simulink model "bh_motor_just_dc_motor_EXPLORE"  (R2017b)
settings: Solver=ode15s  StartTime=0.0  StopTime=30  RelTol=1e-3  EnableMultiTasking=on
undefined symbols (not defined in the file): sigbuilder_block
libraries: fl_lib x30, nesl_utility x20, elec_lib x3
settings Model: Creator=bhorton  LastModifiedBy=bhorton
settings DataIOCC: LimitDataPoints=on
settings OptimizationCC: LifeSpan=inf
settings DebuggingCC: AllowSymbolicDim=off  SFUnexpectedBacktrackingDiag=warning  SFNoUnconditionalDefaultTransitionDiag=warning  SFExecutionAtInitializationDiag=none
settings ModelReferenceCC: PropagateSignalLabelsOutOfModel=off
settings CodeAppCC: StateflowObjectComments=on
settings GRTTargetCC: TargetLangStandard=C89/C90 (ANSI)
settings ConfigComp: CovMetricSettings=dw  CovHtmlReporting=on  CovSaveCumulativeToWorkspaceVar=on  CovSaveSingleToWorkspaceVar=on  CovExternalEMLEnable=off
settings SimscapeCC: SimscapeNormalizeSystem=off  SimscapeLogType=all  SimscapeLogDataHistory=10000  SelectedTab=SimMechanics

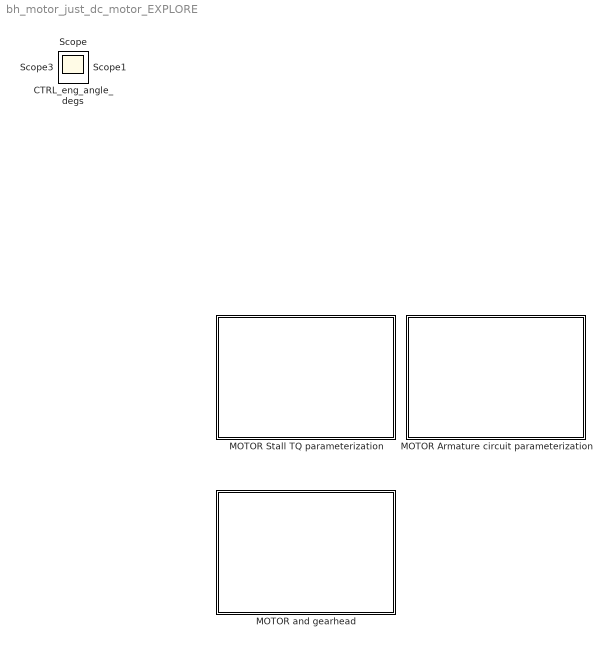
== system bh_motor_just_dc_motor_EXPLORE ==
  MOTOR Armature circuit parameterization : Subsystem
  MOTOR Stall TQ parameterization : Subsystem
  MOTOR and gearhead : Subsystem
  CTRL_eng_angle_degs : Scope
  Scope : Scope
  Scope1 : Scope
  Scope3 : Scope

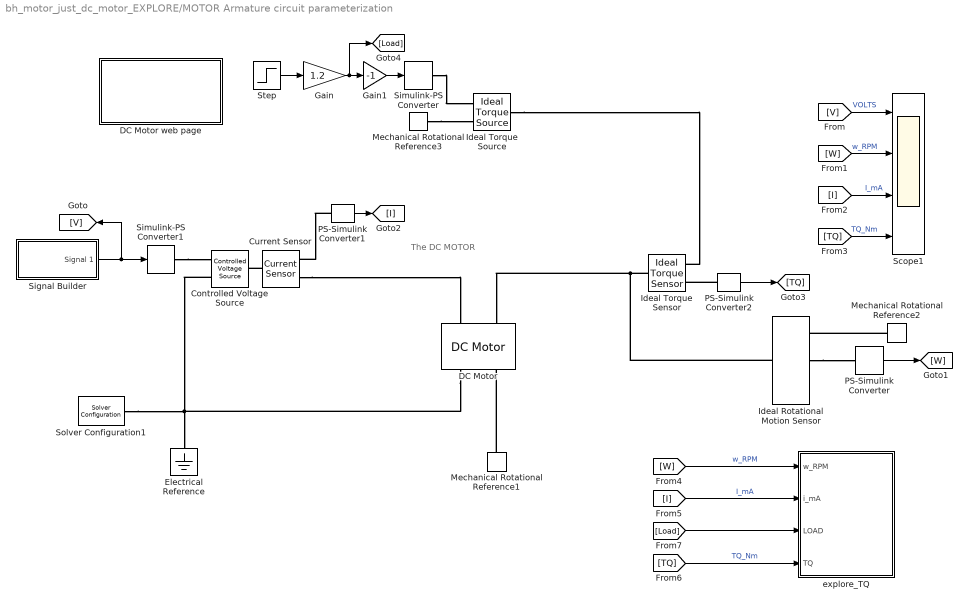
== system bh_motor_just_dc_motor_EXPLORE/MOTOR Armature circuit parameterization ==
  note: The DC MOTOR
  Controlled Voltage Source : fl_lib/Electrical/Electrical Sources/Controlled Voltage Source
  Current Sensor : fl_lib/Electrical/Electrical Sensors/Current Sensor
  DC Motor : elec_lib/Actuators & Drivers/Rotational Actuators/DC Motor  parameterization=1  Ra=5.0117 Ohm  La=1e-4 H  emf_or_torque=2  Kv=7.2e-5 V/rpm  Ki=0.57296 *0.875 N*m/A  T_stall=1.2 N*m  w_max=200 rpm  w_rated=1.5e+4 rpm  P_rated=0.08 W  V_rated=12 V  J=4.5e-5 kg*m^2  lam_param=1  lam=8.20705e-3 N*m/(rad/s)  i_noload=300 mA  V_i_noload=12 V  speed0=0 rpm  alpha=0.00393 1/K  Tmeas=25 C  thermal_mass=100 J/K  initial_temperature=25 C
  DC Motor web page : Subsystem
  Electrical Reference : fl_lib/Electrical/Electrical Elements/Electrical Reference
  Gain : Gain  Gain=1.2
  Gain1 : Gain  Gain=-1
  Ideal Rotational Motion Sensor : fl_lib/Mechanical/Mechanical Sensors/Ideal Rotational Motion Sensor  offset=0 rad
  Ideal Torque Sensor : fl_lib/Mechanical/Mechanical Sensors/Ideal Torque Sensor
  Ideal Torque Source : fl_lib/Mechanical/Mechanical Sources/Ideal Torque Source
  Mechanical Rotational Reference1 : fl_lib/Mechanical/Rotational Elements/Mechanical Rotational Reference
  Mechanical Rotational Reference2 : fl_lib/Mechanical/Rotational Elements/Mechanical Rotational Reference
  Mechanical Rotational Reference3 : fl_lib/Mechanical/Rotational Elements/Mechanical Rotational Reference
  PS-Simulink Converter : nesl_utility/PS-Simulink Converter  PhysicalDomain=network_engine_domain  SubClassName=ps_output  LeftPortType=input  RightPortType=output  PseudoPeriodic=off  Frequencies=[]  Unit=rpm  AffineConversion=off
  PS-Simulink Converter1 : nesl_utility/PS-Simulink Converter  PhysicalDomain=network_engine_domain  SubClassName=ps_output  LeftPortType=input  RightPortType=output  PseudoPeriodic=off  Frequencies=[]  Unit=mA  AffineConversion=off
  PS-Simulink Converter2 : nesl_utility/PS-Simulink Converter  PhysicalDomain=network_engine_domain  SubClassName=ps_output  LeftPortType=input  RightPortType=output  PseudoPeriodic=off  Frequencies=[]  Unit=N*m  AffineConversion=off
  Scope1 : Scope  NumInputPorts=4
  Signal Builder : Subsystem  Tag=STV Subsys  LoadFcn=sigbuilder_block('load');  StartFcn=sigbuilder_block('start');  StopFcn=sigbuilder_block('stop');  ClipboardFcn=sigbuilder_block('clipboard');  mask(Sigbuilder block){tuvar=[0:10]}
      mask help: Simulink:masks:SigbuilderBlock_MD
      mask init:
      | if ~strcmp(get_param(bdroot(gcbh),'SimulationStatus'),'stopped') tuvar = sigbuilder_block('maskInit'); end
      settings: CopyFcn=sigbuilder_block('copy');  DeleteFcn=sigbuilder_block('delete');  ModelCloseFcn=sigbuilder_block('modelClose');  PreSaveFcn=sigbuilder_block('preSave');  PauseFcn=sigbuilder_block('pause');  ContinueFcn=sigbuilder_block('continue');  NameChangeFcn=sigbuilder_block('namechange');  OpenFcn=sigbuilder_block('open',[437.6 199.2 550.4 400 ]);  CloseFcn=sigbuilder_block('close');
      mask Display: plot(0, 0, 100, 100,[2, 2, 32, 32, 2], [68, 8, 8, 68, 68],[32, 2], [38, 38], [32, 19, 2],[53, 60, 44], [32, 17, 17, 2],[16, 16, 31, 31]);txt = getActiveGroup(gcbh);text(2, 100, txt,'verticalAlignment', 'top');
  Simulink-PS Converter : nesl_utility/Simulink-PS Converter  PhysicalDomain=network_engine_domain  SubClassName=ps_input  LeftPortType=input  RightPortType=output  PseudoPeriodic=off  Frequencies=[]  NoiseDistribution=none  NoiseParameters=[]  Unit=N*m  AffineConversion=off  FilteringAndDerivatives=provide  SimscapeFilterOrder=1  InputFilterTimeConstant=0.001  UdotUserProvided=0
  Simulink-PS Converter1 : nesl_utility/Simulink-PS Converter  PhysicalDomain=network_engine_domain  SubClassName=ps_input  LeftPortType=input  RightPortType=output  PseudoPeriodic=off  Frequencies=[]  NoiseDistribution=none  NoiseParameters=[]  Unit=V  AffineConversion=off  FilteringAndDerivatives=zero  SimscapeFilterOrder=1  InputFilterTimeConstant=0.001  UdotUserProvided=1
  Solver Configuration1 : nesl_utility/Solver Configuration  PhysicalDomain=network_engine_domain  SubClassName=solver  LeftPortType=input  RightPortType=generic  Accelerate=off  Tones=[]  Harmonics=[]  SimulateNoise=off  Profile=off  UseLocalSampling=off  EnableSwitchedLinearOptims=on  FrequencyDomain=off  UseCCode=off  RelTol=0.001  AbsTol=1e-06  MinStep=1e-09  ToWorkspace=off  RevertToSquareIcSolve=off  NumHomotopyIterations=100  PhasorMode=off  PhasorModeNumHarmonics=1  DoDC=off  ResidualTolerance=1e-09  UseLocalSolver=off  LocalSolverChoice=NE_BACKWARD_EULER_ADVANCER  LocalSolverSampleTime=0.001  DoFixedCost=off  MaxNonlinIter=3  MaxModeIter=2  LinearAlgebra=Sparse  DelaysMemoryBudget=1024  AutomaticFiltering=on  FilteringTimeConstant=0.001
  Step : Step  Time=25  SampleTime=0
      settings: AttributesFormatString=Step @ t= %<Time>
  explore_TQ : Subsystem
  wires:
  PS-Simulink Converter1/1 -> [I]
  Signal Builder/1(Signal 1) -> [V], Simulink-PS Converter1/1
  [V] -> Scope1/1  "VOLTS"
  [W] -> Scope1/2  "w_RPM"
  [I] -> Scope1/3  "I_mA"
  Step/1 -> Gain/1
  Gain/1 -> [Load], Gain1/1
  PS-Simulink Converter/1 -> [W]
  PS-Simulink Converter2/1 -> [TQ]
  [TQ] -> Scope1/4  "TQ_Nm"
  [TQ] -> explore_TQ/4(TQ)  "TQ_Nm"
  [W] -> explore_TQ/1(w_RPM)  "w_RPM"
  [I] -> explore_TQ/2(i_mA)  "I_mA"
  [Load] -> explore_TQ/3(LOAD)
  Gain1/1 -> Simulink-PS Converter/1
  connections:
  Mechanical Rotational Reference1/LConn1 -- DC Motor/RConn2
  Ideal Rotational Motion Sensor/RConn2 -- PS-Simulink Converter/LConn1
  Mechanical Rotational Reference3/LConn1 -- Ideal Torque Source/RConn2
  Simulink-PS Converter/RConn1 -- Ideal Torque Source/RConn1
  Ideal Torque Source/LConn1 -- Ideal Torque Sensor/RConn1
  Simulink-PS Converter1/RConn1 -- Controlled Voltage Source/RConn1
  Ideal Torque Sensor/LConn1 -- Ideal Rotational Motion Sensor/LConn1 -- DC Motor/LConn2
  Mechanical Rotational Reference2/LConn1 -- Ideal Rotational Motion Sensor/RConn1
  PS-Simulink Converter2/LConn1 -- Ideal Torque Sensor/RConn2
  Controlled Voltage Source/RConn2 -- DC Motor/RConn1 -- Electrical Reference/LConn1 -- Solver Configuration1/RConn1
  PS-Simulink Converter1/LConn1 -- Current Sensor/RConn1
  Current Sensor/RConn2 -- DC Motor/LConn1
  Current Sensor/LConn1 -- Controlled Voltage Source/LConn1

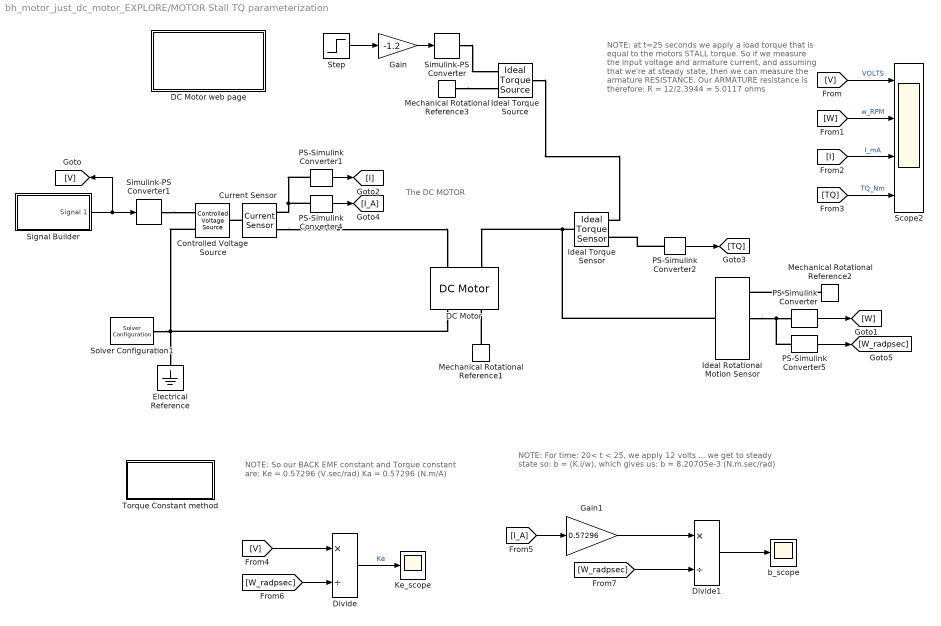
== system bh_motor_just_dc_motor_EXPLORE/MOTOR Stall TQ parameterization ==
  note: The DC MOTOR
  note: NOTE:
      | at t=25 seconds we apply a load torque
      | that is equal to the motors STALL torque.
      |
      | So if we measure the input voltage and armature
      | current, and assuming that we're at steady state,
      | then we can measure the armature RESISTANCE.
      |
      | Our ARMATURE resistance is therefore:
      | R = 12/2.3944 = 5.0117 ohms
  note: NOTE:
      | So our BACK EMF constant and Torque constant are:
      | Ke =  0.57296  (V.sec/rad)
      | Ka =  0.57296  (N.m/A)
  note: NOTE:
      | For time:  20< t < 25, we apply 12 volts ... we get to steady state
      | so:   b = (K.i/w), which gives us:
      | b = 8.20705e-3 (N.m.sec/rad)
  Controlled Voltage Source : fl_lib/Electrical/Electrical Sources/Controlled Voltage Source
  Current Sensor : fl_lib/Electrical/Electrical Sensors/Current Sensor
  DC Motor : elec_lib/Actuators & Drivers/Rotational Actuators/DC Motor  parameterization=2  Ra=2 Ohm  La=1e-4 H  emf_or_torque=2  Kv=7.2e-5 V/rpm  Ki=0.0083 N*m/A  T_stall=1.2 N*m  w_max=200 rpm  w_rated=1.5e+4 rpm  P_rated=0.08 W  V_rated=12 V  J=4.5e-5 kg*m^2  lam_param=2  lam=0.7e-5 N*m/(rad/s)  i_noload=300 mA  V_i_noload=12 V  speed0=0 rpm  alpha=0.00393 1/K  Tmeas=25 C  thermal_mass=100 J/K  initial_temperature=25 C
  DC Motor web page : Subsystem
  Divide : Product  Inputs=*/
  Divide1 : Product  Inputs=*/
  Electrical Reference : fl_lib/Electrical/Electrical Elements/Electrical Reference
  Gain : Gain  Gain=-1.2
  Gain1 : Gain  Gain=0.57296
  Ideal Rotational Motion Sensor : fl_lib/Mechanical/Mechanical Sensors/Ideal Rotational Motion Sensor  offset=0 rad
  Ideal Torque Sensor : fl_lib/Mechanical/Mechanical Sensors/Ideal Torque Sensor
  Ideal Torque Source : fl_lib/Mechanical/Mechanical Sources/Ideal Torque Source
  Ke_scope : Scope
  Mechanical Rotational Reference1 : fl_lib/Mechanical/Rotational Elements/Mechanical Rotational Reference
  Mechanical Rotational Reference2 : fl_lib/Mechanical/Rotational Elements/Mechanical Rotational Reference
  Mechanical Rotational Reference3 : fl_lib/Mechanical/Rotational Elements/Mechanical Rotational Reference
  PS-Simulink Converter : nesl_utility/PS-Simulink Converter  PhysicalDomain=network_engine_domain  SubClassName=ps_output  LeftPortType=input  RightPortType=output  PseudoPeriodic=off  Frequencies=[]  Unit=rpm  AffineConversion=off
  PS-Simulink Converter1 : nesl_utility/PS-Simulink Converter  PhysicalDomain=network_engine_domain  SubClassName=ps_output  LeftPortType=input  RightPortType=output  PseudoPeriodic=off  Frequencies=[]  Unit=mA  AffineConversion=off
  PS-Simulink Converter2 : nesl_utility/PS-Simulink Converter  PhysicalDomain=network_engine_domain  SubClassName=ps_output  LeftPortType=input  RightPortType=output  PseudoPeriodic=off  Frequencies=[]  Unit=N*m  AffineConversion=off
  PS-Simulink Converter4 : nesl_utility/PS-Simulink Converter  PhysicalDomain=network_engine_domain  SubClassName=ps_output  LeftPortType=input  RightPortType=output  PseudoPeriodic=off  Frequencies=[]  Unit=A  AffineConversion=off
  PS-Simulink Converter5 : nesl_utility/PS-Simulink Converter  PhysicalDomain=network_engine_domain  SubClassName=ps_output  LeftPortType=input  RightPortType=output  PseudoPeriodic=off  Frequencies=[]  Unit=rad/s  AffineConversion=off
  Scope2 : Scope  NumInputPorts=4
  Signal Builder : Subsystem  Tag=STV Subsys  LoadFcn=sigbuilder_block('load');  StartFcn=sigbuilder_block('start');  StopFcn=sigbuilder_block('stop');  ClipboardFcn=sigbuilder_block('clipboard');  mask(Sigbuilder block){tuvar=[0:10]}
      mask help: Simulink:masks:SigbuilderBlock_MD
      mask init:
      | if ~strcmp(get_param(bdroot(gcbh),'SimulationStatus'),'stopped') tuvar = sigbuilder_block('maskInit'); end
      settings: CopyFcn=sigbuilder_block('copy');  DeleteFcn=sigbuilder_block('delete');  ModelCloseFcn=sigbuilder_block('modelClose');  PreSaveFcn=sigbuilder_block('preSave');  PauseFcn=sigbuilder_block('pause');  ContinueFcn=sigbuilder_block('continue');  NameChangeFcn=sigbuilder_block('namechange');  OpenFcn=sigbuilder_block('open',[437.6 199.2 550.4 400 ]);  CloseFcn=sigbuilder_block('close');
      mask Display: plot(0, 0, 100, 100,[2, 2, 32, 32, 2], [68, 8, 8, 68, 68],[32, 2], [38, 38], [32, 19, 2],[53, 60, 44], [32, 17, 17, 2],[16, 16, 31, 31]);txt = getActiveGroup(gcbh);text(2, 100, txt,'verticalAlignment', 'top');
  Simulink-PS Converter : nesl_utility/Simulink-PS Converter  PhysicalDomain=network_engine_domain  SubClassName=ps_input  LeftPortType=input  RightPortType=output  PseudoPeriodic=off  Frequencies=[]  NoiseDistribution=none  NoiseParameters=[]  Unit=N*m  AffineConversion=off  FilteringAndDerivatives=provide  SimscapeFilterOrder=1  InputFilterTimeConstant=0.001  UdotUserProvided=0
  Simulink-PS Converter1 : nesl_utility/Simulink-PS Converter  PhysicalDomain=network_engine_domain  SubClassName=ps_input  LeftPortType=input  RightPortType=output  PseudoPeriodic=off  Frequencies=[]  NoiseDistribution=none  NoiseParameters=[]  Unit=V  AffineConversion=off  FilteringAndDerivatives=zero  SimscapeFilterOrder=1  InputFilterTimeConstant=0.001  UdotUserProvided=1
  Solver Configuration1 : nesl_utility/Solver Configuration  PhysicalDomain=network_engine_domain  SubClassName=solver  LeftPortType=input  RightPortType=generic  Accelerate=off  Tones=[]  Harmonics=[]  SimulateNoise=off  Profile=off  UseLocalSampling=off  EnableSwitchedLinearOptims=on  FrequencyDomain=off  UseCCode=off  RelTol=0.001  AbsTol=1e-06  MinStep=1e-09  ToWorkspace=off  RevertToSquareIcSolve=off  NumHomotopyIterations=100  PhasorMode=off  PhasorModeNumHarmonics=1  DoDC=off  ResidualTolerance=1e-09  UseLocalSolver=off  LocalSolverChoice=NE_BACKWARD_EULER_ADVANCER  LocalSolverSampleTime=0.001  DoFixedCost=off  MaxNonlinIter=3  MaxModeIter=2  LinearAlgebra=Sparse  DelaysMemoryBudget=1024  AutomaticFiltering=on  FilteringTimeConstant=0.001
  Step : Step  Time=25  SampleTime=0
      settings: AttributesFormatString=Step @ t= %<Time>
  Torque Constant method : Subsystem
  b_scope : Scope
  wires:
  PS-Simulink Converter1/1 -> [I]
  Signal Builder/1(Signal 1) -> [V], Simulink-PS Converter1/1
  [V] -> Scope2/1  "VOLTS"
  [W] -> Scope2/2  "w_RPM"
  [I] -> Scope2/3  "I_mA"
  Step/1 -> Gain/1
  Gain/1 -> Simulink-PS Converter/1
  PS-Simulink Converter/1 -> [W]
  PS-Simulink Converter2/1 -> [TQ]
  [TQ] -> Scope2/4  "TQ_Nm"
  [V] -> Divide/1
  Divide/1 -> Ke_scope/1  "Ke"
  PS-Simulink Converter4/1 -> [I_A]
  [I_A] -> Gain1/1
  Gain1/1 -> Divide1/1
  PS-Simulink Converter5/1 -> [W_radpsec]
  [W_radpsec] -> Divide/2
  [W_radpsec] -> Divide1/2
  Divide1/1 -> b_scope/1
  connections:
  Mechanical Rotational Reference1/LConn1 -- DC Motor/RConn2
  Ideal Rotational Motion Sensor/RConn2 -- PS-Simulink Converter5/LConn1 -- PS-Simulink Converter/LConn1
  Mechanical Rotational Reference3/LConn1 -- Ideal Torque Source/RConn2
  Simulink-PS Converter/RConn1 -- Ideal Torque Source/RConn1
  Ideal Torque Source/LConn1 -- Ideal Torque Sensor/RConn1
  Simulink-PS Converter1/RConn1 -- Controlled Voltage Source/RConn1
  Ideal Torque Sensor/LConn1 -- Ideal Rotational Motion Sensor/LConn1 -- DC Motor/LConn2
  Mechanical Rotational Reference2/LConn1 -- Ideal Rotational Motion Sensor/RConn1
  PS-Simulink Converter2/LConn1 -- Ideal Torque Sensor/RConn2
  Controlled Voltage Source/RConn2 -- DC Motor/RConn1 -- Electrical Reference/LConn1 -- Solver Configuration1/RConn1
  PS-Simulink Converter1/LConn1 -- PS-Simulink Converter4/LConn1 -- Current Sensor/RConn1
  Current Sensor/RConn2 -- DC Motor/LConn1
  Current Sensor/LConn1 -- Controlled Voltage Source/LConn1

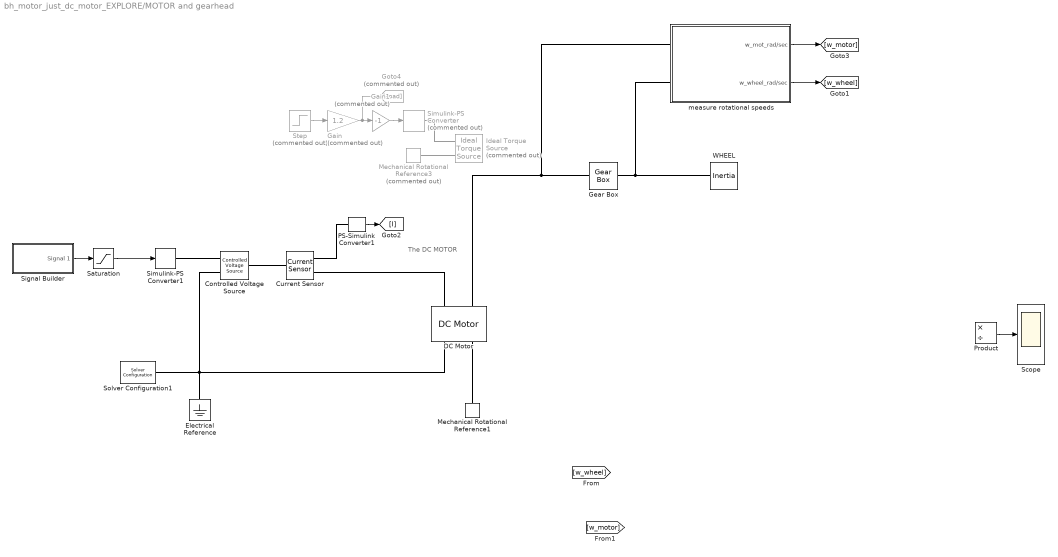
== system bh_motor_just_dc_motor_EXPLORE/MOTOR and gearhead ==
  note: The DC MOTOR
  Controlled Voltage Source : fl_lib/Electrical/Electrical Sources/Controlled Voltage Source
  Current Sensor : fl_lib/Electrical/Electrical Sensors/Current Sensor
  DC Motor : elec_lib/Actuators & Drivers/Rotational Actuators/DC Motor  parameterization=1  Ra=5.0117 Ohm  La=1e-4 H  emf_or_torque=2  Kv=7.2e-5 V/rpm  Ki=0.57296 *0.875 N*m/A  T_stall=1.2 N*m  w_max=200 rpm  w_rated=1.5e+4 rpm  P_rated=0.08 W  V_rated=12 V  J=4.5e-5 kg*m^2  lam_param=1  lam=8.20705e-3 N*m/(rad/s)  i_noload=300 mA  V_i_noload=12 V  speed0=0 rpm  alpha=0.00393 1/K  Tmeas=25 C  thermal_mass=100 J/K  initial_temperature=25 C
  Electrical Reference : fl_lib/Electrical/Electrical Elements/Electrical Reference
  Gain : Gain  Commented=on  Gain=1.2
  Gain1 : Gain  Commented=on  Gain=-1
  Gear Box : fl_lib/Mechanical/Mechanisms/Gear Box  ratio=1  t_in_specify=off  t_in_priority=None  t_in=0 N*m  t_in_nominal_specify=off  t_in_nominal_unit=N*m  t_in_nominal_value=1  t_out_specify=off  t_out_priority=None  t_out=0 N*m  t_out_nominal_specify=off  t_out_nominal_unit=N*m  t_out_nominal_value=1
      settings: AttributesFormatString=|
      | G = (w_in     / w_out)
      | G = (T_out /  T_in)
      | G = %<ratio>
  Goto4 : Goto  Commented=on  GotoTag=Load
  Ideal Torque Source : fl_lib/Mechanical/Mechanical Sources/Ideal Torque Source  Commented=on
  Mechanical Rotational Reference1 : fl_lib/Mechanical/Rotational Elements/Mechanical Rotational Reference
  Mechanical Rotational Reference3 : fl_lib/Mechanical/Rotational Elements/Mechanical Rotational Reference  Commented=on
  PS-Simulink Converter1 : nesl_utility/PS-Simulink Converter  PhysicalDomain=network_engine_domain  SubClassName=ps_output  LeftPortType=input  RightPortType=output  PseudoPeriodic=off  Frequencies=[]  Unit=mA  AffineConversion=off
  Product : Product  Inputs=*/
  Saturation : Saturate
  Scope : Scope  NumInputPorts=3
  Signal Builder : Subsystem  Tag=STV Subsys  LoadFcn=sigbuilder_block('load');  StartFcn=sigbuilder_block('start');  StopFcn=sigbuilder_block('stop');  ClipboardFcn=sigbuilder_block('clipboard');  mask(Sigbuilder block){tuvar=[0:10]}
      mask help: Simulink:masks:SigbuilderBlock_MD
      mask init:
      | if ~strcmp(get_param(bdroot(gcbh),'SimulationStatus'),'stopped') tuvar = sigbuilder_block('maskInit'); end
      settings: CopyFcn=sigbuilder_block('copy');  DeleteFcn=sigbuilder_block('delete');  ModelCloseFcn=sigbuilder_block('modelClose');  PreSaveFcn=sigbuilder_block('preSave');  PauseFcn=sigbuilder_block('pause');  ContinueFcn=sigbuilder_block('continue');  NameChangeFcn=sigbuilder_block('namechange');  OpenFcn=sigbuilder_block('open',[437.6 199.2 550.4 400 ]);  CloseFcn=sigbuilder_block('close');
      mask Display: plot(0, 0, 100, 100,[2, 2, 32, 32, 2], [68, 8, 8, 68, 68],[32, 2], [38, 38], [32, 19, 2],[53, 60, 44], [32, 17, 17, 2],[16, 16, 31, 31]);txt = getActiveGroup(gcbh);text(2, 100, txt,'verticalAlignment', 'top');
  Simulink-PS Converter : nesl_utility/Simulink-PS Converter  Commented=on  PhysicalDomain=network_engine_domain  SubClassName=ps_input  LeftPortType=input  RightPortType=output  PseudoPeriodic=off  Frequencies=[]  NoiseDistribution=none  NoiseParameters=[]  Unit=N*m  AffineConversion=off  FilteringAndDerivatives=provide  SimscapeFilterOrder=1  InputFilterTimeConstant=0.001  UdotUserProvided=0
  Simulink-PS Converter1 : nesl_utility/Simulink-PS Converter  PhysicalDomain=network_engine_domain  SubClassName=ps_input  LeftPortType=input  RightPortType=output  PseudoPeriodic=off  Frequencies=[]  NoiseDistribution=none  NoiseParameters=[]  Unit=V  AffineConversion=off  FilteringAndDerivatives=zero  SimscapeFilterOrder=1  InputFilterTimeConstant=0.001  UdotUserProvided=1
  Solver Configuration1 : nesl_utility/Solver Configuration  PhysicalDomain=network_engine_domain  SubClassName=solver  LeftPortType=input  RightPortType=generic  Accelerate=off  Tones=[]  Harmonics=[]  SimulateNoise=off  Profile=off  UseLocalSampling=off  EnableSwitchedLinearOptims=on  FrequencyDomain=off  UseCCode=off  RelTol=0.001  AbsTol=1e-06  MinStep=1e-09  ToWorkspace=off  RevertToSquareIcSolve=off  NumHomotopyIterations=100  PhasorMode=off  PhasorModeNumHarmonics=1  DoDC=off  ResidualTolerance=1e-09  UseLocalSolver=off  LocalSolverChoice=NE_BACKWARD_EULER_ADVANCER  LocalSolverSampleTime=0.001  DoFixedCost=off  MaxNonlinIter=3  MaxModeIter=2  LinearAlgebra=Sparse  DelaysMemoryBudget=1024  AutomaticFiltering=on  FilteringTimeConstant=0.001
  Step : Step  Commented=on  Time=25  SampleTime=0
      settings: AttributesFormatString=Step @ t= %<Time>
  WHEEL : fl_lib/Mechanical/Rotational Elements/Inertia  inertia=0.01 kg*m^2  w_specify=off  w_priority=High  w=0 rad/s  w_nominal_specify=off  w_nominal_unit=rad/s  w_nominal_value=1  t_specify=off  t_priority=None  t=0 N*m  t_nominal_specify=off  t_nominal_unit=N*m  t_nominal_value=1
  measure rotational speeds : Subsystem
  wires:
  PS-Simulink Converter1/1 -> [I]
  Signal Builder/1(Signal 1) -> Saturation/1
  Step/1 -> Gain/1
  Gain/1 -> Goto4/1, Gain1/1
  Gain1/1 -> Simulink-PS Converter/1
  Product/1 -> Scope/2
  Saturation/1 -> Simulink-PS Converter1/1
  measure rotational speeds/2(w_wheel_rad/sec) -> [w_wheel]
  measure rotational speeds/1(w_mot_rad/sec) -> [w_motor]
  connections:
  Mechanical Rotational Reference1/LConn1 -- DC Motor/RConn2
  Mechanical Rotational Reference3/LConn1 -- Ideal Torque Source/RConn2
  Simulink-PS Converter/RConn1 -- Ideal Torque Source/RConn1
  Simulink-PS Converter1/RConn1 -- Controlled Voltage Source/RConn1
  Controlled Voltage Source/RConn2 -- DC Motor/RConn1 -- Solver Configuration1/RConn1 -- Electrical Reference/LConn1
  PS-Simulink Converter1/LConn1 -- Current Sensor/RConn1
  Current Sensor/RConn2 -- DC Motor/LConn1
  Current Sensor/LConn1 -- Controlled Voltage Source/LConn1
  Gear Box/LConn1 -- measure rotational speeds/LConn1 -- DC Motor/LConn2
  WHEEL/LConn1 -- measure rotational speeds/LConn2 -- Gear Box/RConn1

== system bh_motor_just_dc_motor_EXPLORE/MOTOR Armature circuit parameterization/DC Motor web page ==
  note: http://www.onlineconversion.com/torque.htm
  note: 170 ounce inch = 1.2004638117 newton meter
  note: 50:1 powerful brushed DC motor
      | Speed (no load): 200RPM (12V)
      | Stall torque: 170 oz·in (12V)
      | Free-run current (no load): 300 mA (12V)
  note: http://www.robotshop.com/en/12v-501-170oz-inc-metal-gearmotor.html

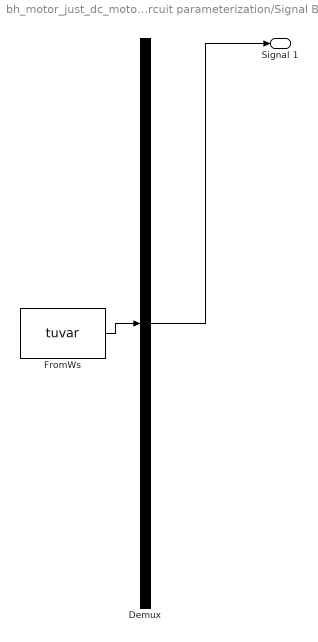
== system bh_motor_just_dc_motor_EXPLORE/MOTOR Armature circuit parameterization/Signal Builder ==
  Demux : Demux  Tag=STV Demux  Outputs=1
  FromWs : FromWorkspace  Tag=STV FromWs  VariableName=tuvar  SampleTime=0
      SigBuilderData=|
      | common.afterFinalStr = 'Extrapolate'
      | common.sampleTime = 0
      | dataSet.timeRange = [0 30]
      | dataSet.name = 'Group 1'
      | sbobj.Groups.Name = 'Group 1'
      | sbobj.Groups.Signals.Name = 'Signal 1'
      | sbobj.Groups.Signals.XData = [0 5.05 5.05 10 10 15.05 15.05 20 20 24.95 30]
      | sbobj.Groups.Signals.YData = [1 1 3 3 6 6 9 9 12 12 12]
      | sbobj.Groups.TimeRange = [0 30]
  Signal 1 : Outport  Tag=STV Outport
  wires:
  Demux/1 -> Signal 1/1
  FromWs/1 -> Demux/1

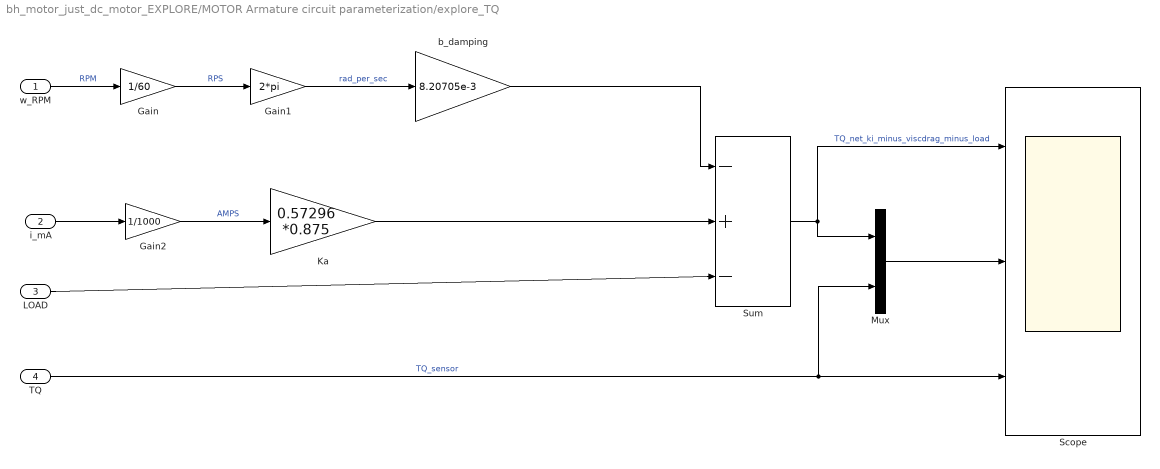
== system bh_motor_just_dc_motor_EXPLORE/MOTOR Armature circuit parameterization/explore_TQ ==
  w_RPM : Inport
  i_mA : Inport  Port=2
  LOAD : Inport  Port=3
  TQ : Inport  Port=4
  Gain : Gain  Gain=1/60
  Gain1 : Gain  Gain=2*pi
  Gain2 : Gain  Gain=1/1000
  Ka : Gain  Gain=0.57296 *0.875
  Mux : Mux  Inputs=2
  Scope : Scope  NumInputPorts=3
  Sum : Sum  Inputs=-|+|-
  b_damping : Gain  Gain=8.20705e-3
  wires:
  w_RPM/1 -> Gain/1  "RPM"
  Gain/1 -> Gain1/1  "RPS"
  Gain1/1 -> b_damping/1  "rad_per_sec"
  i_mA/1 -> Gain2/1
  b_damping/1 -> Sum/1
  Ka/1 -> Sum/2
  Sum/1 -> Scope/1, Mux/1  "TQ_net_ki_minus_viscdrag_minus_load"
  TQ/1 -> Scope/3, Mux/2  "TQ_sensor"
  Gain2/1 -> Ka/1  "AMPS"
  Mux/1 -> Scope/2
  LOAD/1 -> Sum/3

== system bh_motor_just_dc_motor_EXPLORE/MOTOR Stall TQ parameterization/DC Motor web page ==
  note: http://www.onlineconversion.com/torque.htm
  note: 170 ounce inch = 1.2004638117 newton meter
  note: 50:1 powerful brushed DC motor
      | Speed (no load): 200RPM (12V)
      | Stall torque: 170 oz·in (12V)
      | Free-run current (no load): 300 mA (12V)
  note: http://www.robotshop.com/en/12v-501-170oz-inc-metal-gearmotor.html

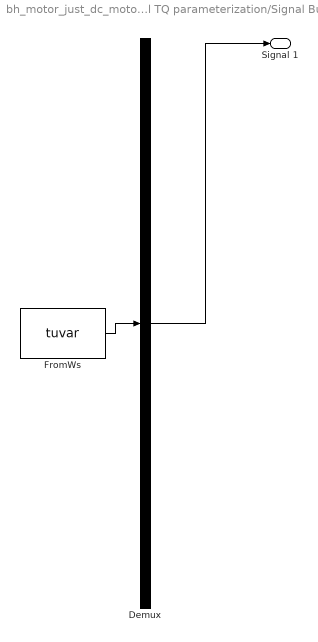
== system bh_motor_just_dc_motor_EXPLORE/MOTOR Stall TQ parameterization/Signal Builder ==
  Demux : Demux  Tag=STV Demux  Outputs=1
  FromWs : FromWorkspace  Tag=STV FromWs  VariableName=tuvar  SampleTime=0
      SigBuilderData=|
      | common.afterFinalStr = 'Extrapolate'
      | common.sampleTime = 0
      | dataSet.timeRange = [0 30]
      | dataSet.name = 'Group 1'
      | sbobj.Groups.Name = 'Group 1'
      | sbobj.Groups.Signals.Name = 'Signal 1'
      | sbobj.Groups.Signals.XData = [0 5.05 5.05 10 10 15.05 15.05 20 20 24.95 30]
      | sbobj.Groups.Signals.YData = [1 1 3 3 6 6 9 9 12 12 12]
      | sbobj.Groups.TimeRange = [0 30]
  Signal 1 : Outport  Tag=STV Outport
  wires:
  Demux/1 -> Signal 1/1
  FromWs/1 -> Demux/1

== system bh_motor_just_dc_motor_EXPLORE/MOTOR Stall TQ parameterization/Torque Constant method ==

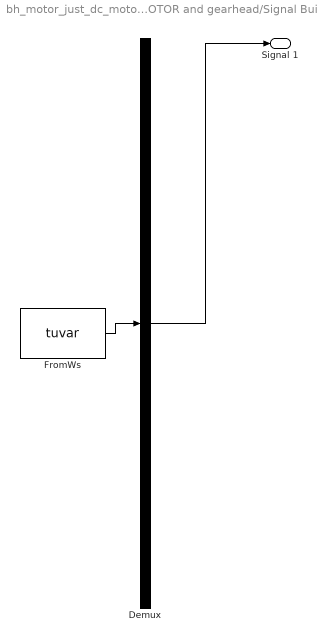
== system bh_motor_just_dc_motor_EXPLORE/MOTOR and gearhead/Signal Builder ==
  Demux : Demux  Tag=STV Demux  Outputs=1
  FromWs : FromWorkspace  Tag=STV FromWs  VariableName=tuvar  SampleTime=0
      SigBuilderData=|
      | common.afterFinalStr = 'Extrapolate'
      | common.sampleTime = 0
      | dataSet.timeRange = [0 30]
      | dataSet.name = 'Group 1'
      | sbobj.Groups.Name = 'Group 1'
      | sbobj.Groups.Signals.Name = 'Signal 1'
      | sbobj.Groups.Signals.XData = [0 5.05 5.05 10 10 15.05 15.05 20 20 24.95 30]
      | sbobj.Groups.Signals.YData = [1 1 3 3 6 6 9 9 12 12 12]
      | sbobj.Groups.TimeRange = [0 30]
  Signal 1 : Outport  Tag=STV Outport
  wires:
  Demux/1 -> Signal 1/1
  FromWs/1 -> Demux/1

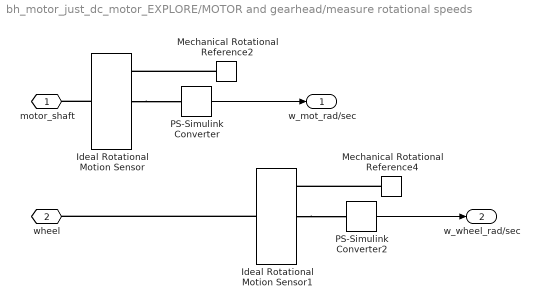
== system bh_motor_just_dc_motor_EXPLORE/MOTOR and gearhead/measure rotational speeds ==
  Ideal Rotational Motion Sensor : fl_lib/Mechanical/Mechanical Sensors/Ideal Rotational Motion Sensor  offset=0 rad
  Ideal Rotational Motion Sensor1 : fl_lib/Mechanical/Mechanical Sensors/Ideal Rotational Motion Sensor  offset=0 rad
  Mechanical Rotational Reference2 : fl_lib/Mechanical/Rotational Elements/Mechanical Rotational Reference
  Mechanical Rotational Reference4 : fl_lib/Mechanical/Rotational Elements/Mechanical Rotational Reference
  PS-Simulink Converter : nesl_utility/PS-Simulink Converter  PhysicalDomain=network_engine_domain  SubClassName=ps_output  LeftPortType=input  RightPortType=output  PseudoPeriodic=off  Frequencies=[]  Unit=rad/s  AffineConversion=off
  PS-Simulink Converter2 : nesl_utility/PS-Simulink Converter  PhysicalDomain=network_engine_domain  SubClassName=ps_output  LeftPortType=input  RightPortType=output  PseudoPeriodic=off  Frequencies=[]  Unit=rad/s  AffineConversion=off
  motor_shaft : PMIOPort  Port=1  Side=Left
  wheel : PMIOPort  Port=2  Side=Left
  w_mot_rad/sec : Outport
  w_wheel_rad/sec : Outport  Port=2
  wires:
  PS-Simulink Converter/1 -> w_mot_rad/sec/1
  PS-Simulink Converter2/1 -> w_wheel_rad/sec/1
  connections:
  Ideal Rotational Motion Sensor/RConn2 -- PS-Simulink Converter/LConn1
  Mechanical Rotational Reference2/LConn1 -- Ideal Rotational Motion Sensor/RConn1
  Ideal Rotational Motion Sensor/LConn1 -- motor_shaft/RConn1
  Ideal Rotational Motion Sensor1/LConn1 -- wheel/RConn1
  Mechanical Rotational Reference4/LConn1 -- Ideal Rotational Motion Sensor1/RConn1
  Ideal Rotational Motion Sensor1/RConn2 -- PS-Simulink Converter2/LConn1
